simulink model "Team2_PowerLine_Model_v05"  (R2026a)
settings: Solver=VariableStepAuto  StopTime=0.1  MaxStep=1e-4
libraries: simulink x5
settings Model: Creator=ruyxv  LastModifiedBy=ruyxv

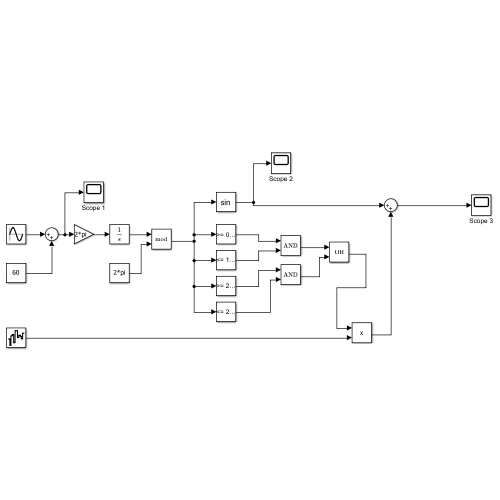
[thumbnail: Simulink's stored preview of the top-level diagram]
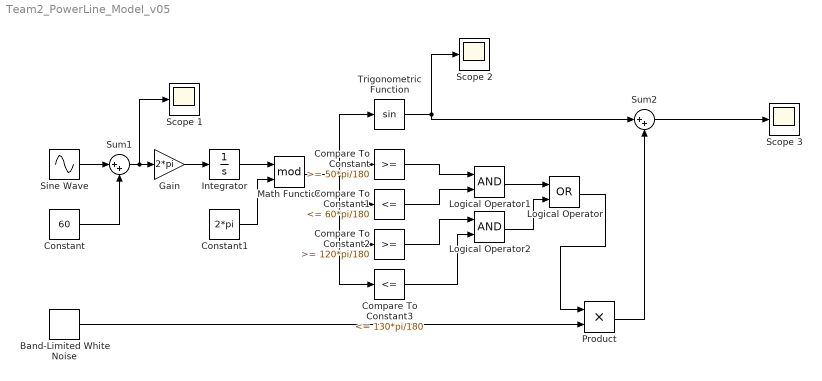
== system Team2_PowerLine_Model_v05 ==
  Band-Limited White Noise : simulink/Sources/Band-Limited White Noise  Cov=1e-5  Ts=1e-4  seed=[23341]
  Compare To Constant : simulink/Logic and Bit Operations/Compare To Constant  relop=>=  const=50*pi/180  OutDataTypeStr=boolean
  Compare To Constant1 : simulink/Logic and Bit Operations/Compare To Constant  relop=<=  const=60*pi/180  OutDataTypeStr=boolean
  Compare To Constant2 : simulink/Logic and Bit Operations/Compare To Constant  relop=>=  const=120*pi/180  OutDataTypeStr=boolean
  Compare To Constant3 : simulink/Logic and Bit Operations/Compare To Constant  relop=<=  const=130*pi/180  OutDataTypeStr=boolean
  Constant : Constant  Value=60
  Constant1 : Constant  Value=2*pi
  Gain : Gain  Gain=2*pi
  Integrator : Integrator
  Logical Operator : Logic  Operator=OR  AllPortsSameDT=off  OutDataTypeStr=boolean
  Logical Operator1 : Logic  AllPortsSameDT=off  OutDataTypeStr=boolean
  Logical Operator2 : Logic  AllPortsSameDT=off  OutDataTypeStr=boolean
  Math Function : Math  Operator=mod
  Product : Product
  Scope 1 : Scope
      settings: ActiveDisplayYMinimum=59.975000000035017  ActiveDisplayYMaximum=60.02499999996499
  Scope 2 : Scope
      settings: ActiveDisplayYMinimum=-1  ActiveDisplayYMaximum=1
  Scope 3 : Scope
      settings: ActiveDisplayYMinimum=-1.2870754699674019  ActiveDisplayYMaximum=1.583679234461697  DataLoggingVariableName=ScopeData2
  Sine Wave : Sin  Amplitude=0.02  Frequency=2*pi*0.5  SampleTime=0
  Sum1 : Sum  Inputs=|++
  Sum2 : Sum  Inputs=|++
  Trigonometric Function : Trigonometry
  wires:
  Sine Wave/1 -> Sum1/1
  Gain/1 -> Integrator/1
  Constant/1 -> Sum1/2
  Sum1/1 -> Scope 1/1, Gain/1
  Band-Limited White Noise/1 -> Product/2
  Sum2/1 -> Scope 3/1
  Product/1 -> Sum2/2
  Logical Operator2/1 -> Logical Operator/2
  Logical Operator1/1 -> Logical Operator/1
  Logical Operator/1 -> Product/1
  Trigonometric Function/1 -> Scope 2/1, Sum2/1
  Compare To Constant/1 -> Logical Operator1/1
  Compare To Constant1/1 -> Logical Operator1/2
  Compare To Constant2/1 -> Logical Operator2/1
  Compare To Constant3/1 -> Logical Operator2/2
  Math Function/1 -> Compare To Constant3/1, Compare To Constant2/1, Compare To Constant1/1, Compare To Constant/1, Trigonometric Function/1
  Integrator/1 -> Math Function/1
  Constant1/1 -> Math Function/2
